simulink model "MdEnChk6s7s_EZE"  (R2018b)
settings: Solver=FixedStepDiscrete  StartTime=0.0  StopTime=10.0  FixedStep=0.01  RelTol=1e-3
undefined symbols (not defined in the file or in its folder): IsStBsy32_Set, ModeState32_Set, SetBit
settings Model: Creator=sn2xws  LastModifiedBy=sn2xws
settings DataIOCC: SaveFormat=StructureWithTime
settings OptimizationCC: DefaultParameterBehavior=Inlined  EnhancedBackFolding=on  PassReuseOutputArgsAs=Individual arguments  ZeroExternalMemoryAtStartup=off  ZeroInternalMemoryAtStartup=off  OptimizeBlockOrder=speed  DifferentSizesBufferReuse=on  OptimizationCustomize=off
settings DebuggingCC: ParameterTunabilityLossMsg=error
settings ModelReferenceCC: ModelReferenceNumInstancesAllowed=Single
settings SFSimCC: MATLABDynamicMemAlloc=off
settings RTWCC: SystemTargetFile=autosar.tlc  GenCodeOnly=on  TemplateMakefile=ert_default_tmf  Description=AUTOSAR  GenerateReport=on  IncludeHyperlinkInReport=on  LaunchReport=on  GenerateTraceInfo=on  GenerateTraceReport=on  GenerateTraceReportSl=on  GenerateTraceReportSf=on  GenerateTraceReportEml=on  GenerateCodeMetricsReport=on
settings CodeAppCC: ForceParamTrailComments=on  IgnoreCustomStorageClasses=off  OperatorAnnotations=on  SimulinkDataObjDesc=on  SFDataObjDesc=on  InsertBlockDesc=on
settings STFCustomTargetCC: TargetLangStandard=C99 (ISO)  MultiwordLength=256  ParMdlRefBuildCompliant=on  CompOptLevelCompliant=on  IncludeMdlTerminateFcn=off  CombineOutputUpdateFcns=on  SuppressErrorStatus=on  ERTCustomFileBanners=on  SupportNonFinite=off  SupportComplex=off  SupportContinuousTime=off  SupportNonInlinedSFcns=off  RemoveResetFunc=on  MATLABClassNameForMDSCustomization=Simulink.SoftwareTarget.ERTCustomization  AutosarCompliant=on  UseToolchainInfoCompliant=on  LookupTableObjectStructAxisOrder=2,1,3,4,...  LUTObjectStructOrderEvenSpacing=Size,Table,Breakpoints  SystemTargetFile=autosar.tlc
settings ERTTargetCC: TargetLangStandard=C99 (ISO)  ConcurrentExecutionCompliant=off  IncludeMdlTerminateFcn=off  SuppressErrorStatus=on  SupportNonFinite=off  SupportComplex=off  ModelStepFunctionPrototypeControlCompliant=off  CPPClassGenCompliant=off  AutosarCompliant=on  LookupTableObjectStructAxisOrder=2,1,3,4,...  LUTObjectStructOrderEvenSpacing=Size,Table,Breakpoints  InlinedParameterPlacement=NonHierarchical  ERTCustomFileTemplate=example_file_process.tlc

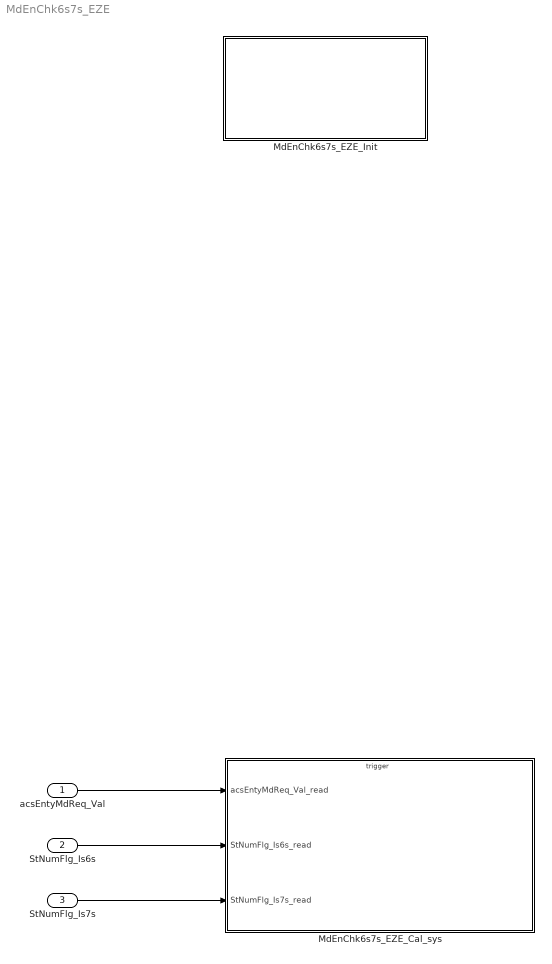
== system MdEnChk6s7s_EZE ==
  acsEntyMdReq_Val : Inport  OutDataTypeStr=boolean  PortDimensions=1
  StNumFlg_Is6s : Inport  Port=2  OutDataTypeStr=boolean  PortDimensions=1
  StNumFlg_Is7s : Inport  Port=3  OutDataTypeStr=boolean  PortDimensions=1
  MdEnChk6s7s_EZE_Cal_sys : Subsystem
  MdEnChk6s7s_EZE_Init : Subsystem
  wires:
  acsEntyMdReq_Val/1 -> MdEnChk6s7s_EZE_Cal_sys/1(acsEntyMdReq_Val_read)
  StNumFlg_Is7s/1 -> MdEnChk6s7s_EZE_Cal_sys/3(StNumFlg_Is7s_read)
  StNumFlg_Is6s/1 -> MdEnChk6s7s_EZE_Cal_sys/2(StNumFlg_Is6s_read)

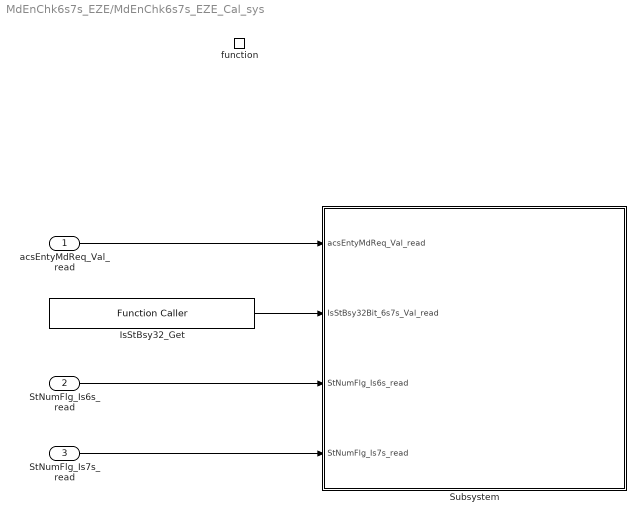
== system MdEnChk6s7s_EZE/MdEnChk6s7s_EZE_Cal_sys ==
  acsEntyMdReq_Val_read : Inport
  StNumFlg_Is6s_read : Inport  Port=2
  StNumFlg_Is7s_read : Inport  Port=3
  function : TriggerPort  TriggerType=function-call  IsSimulinkFunction=on  FunctionName=MdEnChk6s7s_EZE_Cal  VariantControl=(inherit)
  IsStBsy32_Get : FunctionCaller  FunctionPrototype=IsStBsy32Bit = IsStBsy32_Get()  OutputArgumentSpecifications=uint32(1)
  Subsystem : Subsystem
  wires:
  acsEntyMdReq_Val_read/1 -> Subsystem/1(acsEntyMdReq_Val_read)
  StNumFlg_Is6s_read/1 -> Subsystem/3(StNumFlg_Is6s_read)
  StNumFlg_Is7s_read/1 -> Subsystem/4(StNumFlg_Is7s_read)
  IsStBsy32_Get/1 -> Subsystem/2(IsStBsy32Bit_6s7s_Val_read)

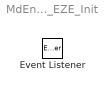
== system MdEnChk6s7s_EZE/MdEnChk6s7s_EZE_Init ==
  Event Listener : EventListener  EventName=reset

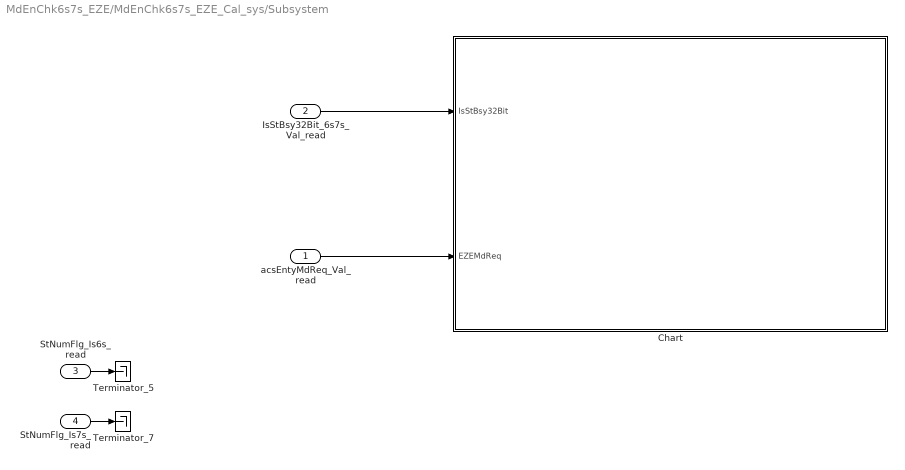
== system MdEnChk6s7s_EZE/MdEnChk6s7s_EZE_Cal_sys/Subsystem ==
  acsEntyMdReq_Val_read : Inport
  IsStBsy32Bit_6s7s_Val_read : Inport  Port=2
  StNumFlg_Is6s_read : Inport  Port=3
  StNumFlg_Is7s_read : Inport  Port=4
  Chart : Stateflow chart  TreatAsAtomicUnit=on
  Terminator_5 : Terminator
  Terminator_7 : Terminator
  wires:
  StNumFlg_Is7s_read/1 -> Terminator_7/1
  StNumFlg_Is6s_read/1 -> Terminator_5/1
  acsEntyMdReq_Val_read/1 -> Chart/2(EZEMdReq)
  IsStBsy32Bit_6s7s_Val_read/1 -> Chart/1(IsStBsy32Bit)

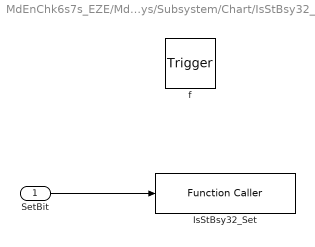
== system MdEnChk6s7s_EZE/MdEnChk6s7s_EZE_Cal_sys/Subsystem/Chart/IsStBsy32_Set ==
  SetBit : Inport
  f : TriggerPort  TriggerType=function-call  VariantControl=(inherit)
      settings: CopyFcn=Stateflow.SLINSF.SimulinkMan.removeBlockPreDeleteFcn  PreDeleteFcn=Stateflow.SLINSF.SimulinkMan.unsafePredeleteFcn
  IsStBsy32_Set : FunctionCaller  FunctionPrototype=IsStBsy32_Set(SetBit)  InputArgumentSpecifications=uint32(1)
  wires:
  SetBit/1 -> IsStBsy32_Set/1

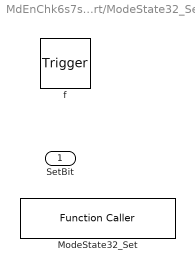
== system MdEnChk6s7s_EZE/MdEnChk6s7s_EZE_Cal_sys/Subsystem/Chart/ModeState32_Set ==
  SetBit : Inport
  f : TriggerPort  TriggerType=function-call  VariantControl=(inherit)
      settings: CopyFcn=Stateflow.SLINSF.SimulinkMan.removeBlockPreDeleteFcn  PreDeleteFcn=Stateflow.SLINSF.SimulinkMan.unsafePredeleteFcn
  ModeState32_Set : FunctionCaller  FunctionPrototype=ModeState32_Set(SetBit)  InputArgumentSpecifications=uint32(1)

== stateflow chart MdEnChk6s7s_EZE/MdEnChk6s7s_EZE_Cal_sys/Subsystem/Chart ==
  state IsStBsy32_Set(SetBit) [function]
  state ModeState32_Set(SetBit) [function]
  (default) -> (junction 252)
  (junction 252) -> (junction 249) [order 1] : [hasChangedTo(EZEMdReq,true)&&((IsStBsy32Bit&EZEBit)==0)]
  (junction 252) -> (junction 251) [order 2]
  (junction 249) -> (junction 250) : {
      | ModeState32_Set(EZEBit);
      | BsySetBit = (EZEBit+EZQBit+VIPLBit+VIPRBit+VIPAllBit+RcvyLBit+RcvyRBit+LugLBit+LugRBit+LugAllBit+FamlyLBit+FamlyRBit+INTMLBit+INTMRBit);
      | IsStBsy32_Set(BsySetBit);
      | }
  (junction 250) -> (junction 251)
  (junction 251) -> (junction 258)
  data: SetBit function_input; SetBit function_input; IsStBsy32Bit input uint32; EZEBit constant uint32 =1; EZQBit constant uint32 =8; VIPAllBit constant uint32 =2; LugAllBit constant uint32 =4; VIPLBit constant uint32 =512; VIPRBit constant uint32 =2048; RcvyLBit constant uint32 =1024; RcvyRBit constant uint32 =4096; INTMLBit constant uint32 =16; INTMRBit constant uint32 =524288; FamlyLBit constant uint32 =64; FamlyRBit constant uint32 =32; LugLBit constant uint32 =128; LugRBit constant uint32 =256; EZEMdReq input; BsySetBit local uint32
